simulink model "simulacao_controlador_perturbacao"  (R2018b)
settings: Solver=VariableStepAuto  StartTime=0.0  StopTime=3000  RelTol=1e-3
undefined symbols (not defined in the file): sp_h3, sp_h4, sp_u, T
settings Model: Creator=tarsis  LastModifiedBy=tarsis

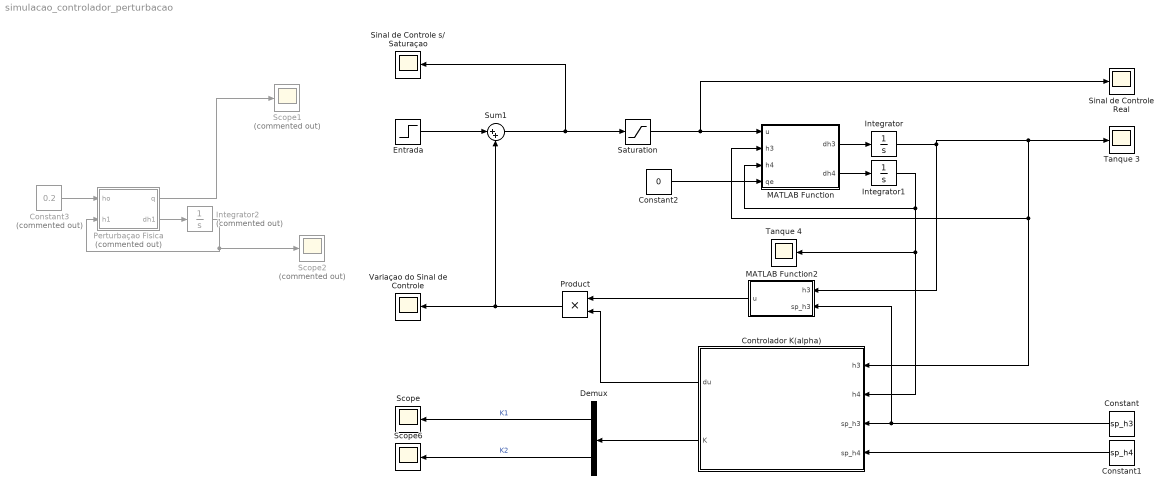
== system simulacao_controlador_perturbacao ==
  Constant : Constant  Value=sp_h3
  Constant1 : Constant  Value=sp_h4
  Constant2 : Constant  Value=0
  Constant3 : Constant  Commented=on  Value=0.2
  Controlador K(alpha) : MATLAB Function  TreatAsAtomicUnit=on
  Demux : Demux  Outputs=2
  Entrada : Step  Time=0  After=sp_u  SampleTime=T
  Integrator : Integrator
  Integrator1 : Integrator
  Integrator2 : Integrator  Commented=on
  MATLAB Function : MATLAB Function  TreatAsAtomicUnit=on
  MATLAB Function2 : MATLAB Function  TreatAsAtomicUnit=on
  Perturbaçao Fisica : MATLAB Function  Commented=on  TreatAsAtomicUnit=on
  Product : Product
  Saturation : Saturate  UpperLimit=60  LowerLimit=0
  Scope : Scope
  Scope1 : Scope  Commented=on
  Scope2 : Scope  Commented=on
  Scope6 : Scope
  Sinal de Controle Real : Scope
  Sinal de Controle s/ Saturaçao : Scope
  Sum1 : Sum  Inputs=|++
  Tanque 3 : Scope
  Tanque 4 : Scope
  "Variaçao do Sinal de Controle " : Scope
  wires:
  Integrator/1 -> Controlador K(alpha)/1(h3), MATLAB Function/2(h3), Tanque 3/1, MATLAB Function2/1(h3)
  Product/1 -> Sum1/2, "Variaçao do Sinal de Controle "/1
  MATLAB Function2/1(u) -> Product/1
  Demux/1 -> Scope/1  "K1"
  Sum1/1 -> Sinal de Controle s/ Saturaçao/1, Saturation/1
  Integrator1/1 -> Controlador K(alpha)/2(h4), Tanque 4/1, MATLAB Function/3(h4)
  Controlador K(alpha)/1(du) -> Product/2
  Constant/1 -> MATLAB Function2/2(sp_h3), Controlador K(alpha)/3(sp_h3)
  Demux/2 -> Scope6/1  "K2"
  MATLAB Function/2(dh4) -> Integrator1/1
  Entrada/1 -> Sum1/1
  Controlador K(alpha)/2(K) -> Demux/1
  Saturation/1 -> Sinal de Controle Real/1, MATLAB Function/1(u)
  Constant1/1 -> Controlador K(alpha)/4(sp_h4)
  MATLAB Function/1(dh3) -> Integrator/1
  Constant2/1 -> MATLAB Function/4(qe)
  Constant3/1 -> Perturbaçao Fisica/1(ho)
  Perturbaçao Fisica/1(q) -> Scope1/1
  Integrator2/1 -> Perturbaçao Fisica/2(h1), Scope2/1
  Perturbaçao Fisica/2(dh1) -> Integrator2/1

== matlab function simulacao_controlador_perturbacao/Controlador K(alpha) ==
  data: h3 input; du output; h4 input; sp_h3 input; sp_h4 input; K output
function [du,K] = fcn(h3,h4,sp_h3,sp_h4)
h = [h4 h3]';
sp_h = [sp_h4 sp_h3]';
K1 = [-3.137 -1.8025]*1e3;
K2 = [-3.1370 -1.5129]*1e3;
K = h3*0.05*(K2 - K1) + 2.4*K1 - 1.4*K2;
du = K*(h - sp_h);

== matlab function simulacao_controlador_perturbacao/MATLAB Function ==
  data: u input; dh3 output; dh4 output; h3 input; h4 input; qe input
function [dh3,dh4] = fcn(u,h3,h4,qe)
qi = (16.4*u + 357.3)*1e-6;
q12 = 33.51e-4*(h4 - h3) + 43.12e-5;
qout = (87.07e-5*sqrt(h3) + 30.99e-5);
A1 = (pi*(31)^2)*1e-4;
A2 = - 0.88629272879272778105782609278436*h3^16 + 6.0267905557905489111932174309337*h3^15 - 20.80464391736738395516887057851*h3^14 + 47.68494439008527766774004035511*h3^13 - 82.573907447205791291786792565001*h3^12 + 116.28257881925208875326233578017*h3^11 - 139.30893428077013388311346843447*h3^10 + 144.80767028205944702410747888441*h3^9 - 129.2475129476872169884635810807*h3^8 + 96.099152680911332924853135955618*h3^7 - 55.593870964701796673125553833866*h3^6 + 21.451550218200266654046211819752*h3^5 - 5.9275208717979510465216954484015*h3^4 + 3.9856416105248966168880953176109*h3^3 - 2.0902185091906828919771687989635*h3^2 - 0.061481774188906647716430580264178*h3 + 0.32722421068834535751546101783638;
dh4 = (qi - q12)/A1;
dh3 = (q12 - qout + qe)/A2;

== matlab function simulacao_controlador_perturbacao/MATLAB Function2 ==
  settings: updateMethod=DISCRETE
  data: h3 input; u output; sp_h3 input
function u = fcn(h3,sp_h3)

persistent s
if isempty(s)
    s = false;
end

if h3<sp_h3*0.8 && s==false
    u = 0;
else
    u = 1;
    s = true;
end

== matlab function simulacao_controlador_perturbacao/Perturbaçao Fisica ==
  settings: updateMethod=DISCRETE
  data: ho input; q output; h1 input; dh1 output
function [q,dh1] = fcn(ho,h1)
A = (31e-2)^2*pi;
a = (0.3175e-2)^2*pi;
g = 9.81;
persistent h
if isempty(h)
    h1 = ho;
end
h = h1;
q = a*sqrt(2*g*h1);
dh1 = -q/A;
